simulink model "Assemble_Blocks_May_7_2020"  (R2020a)
settings: Solver=VariableStepAuto  StartTime=0.0  StopTime=100  RelTol=1e-3
libraries: sailbot_library x19
settings Model: Creator=tylerlum  LastModifiedBy=Nicolas
settings SFSimCC: CustomCodeUndefinedFunction=UseInterfaceOnly

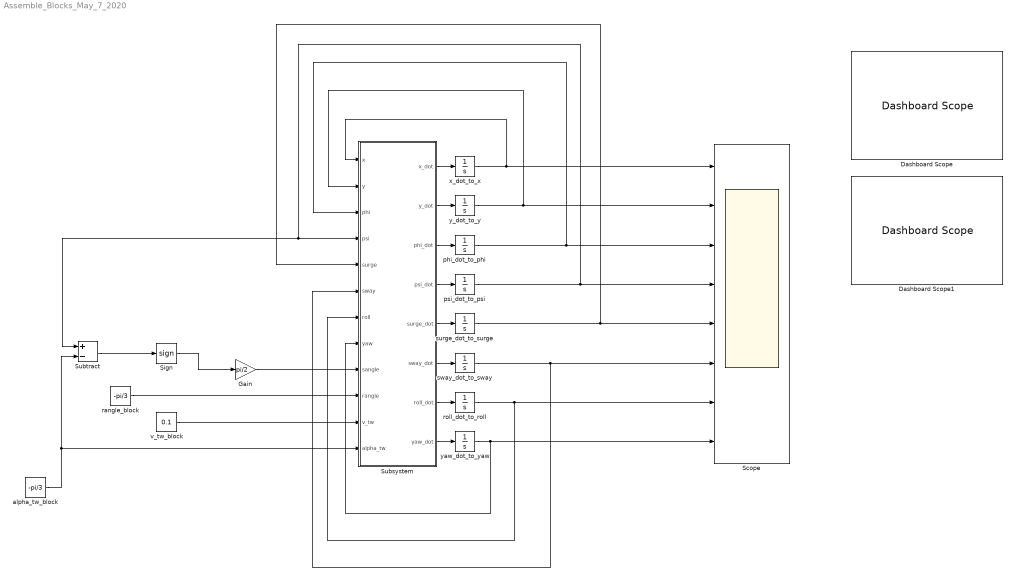
== system Assemble_Blocks_May_7_2020 ==
  Dashboard Scope : DashboardScope
  Dashboard Scope1 : DashboardScope
  Gain : Gain  Gain=pi/2
  Scope : Scope  NumInputPorts=8
  Sign : Signum
  Subsystem : Subsystem
  Subtract : Sum  Inputs=+-
  alpha_tw_block : Constant  Value=-pi/3
  phi_dot_to_phi : Integrator
  psi_dot_to_psi : Integrator  InitialCondition=pi/2
  rangle_block : Constant  Value=-pi/3
  roll_dot_to_roll : Integrator
  surge_dot_to_surge : Integrator
  sway_dot_to_sway : Integrator
  v_tw_block : Constant  Value=0.1
  x_dot_to_x : Integrator
  y_dot_to_y : Integrator
  yaw_dot_to_yaw : Integrator
  wires:
  Subsystem/1(x_dot) -> x_dot_to_x/1
  x_dot_to_x/1 -> Scope/1, Subsystem/1(x)
  Subsystem/2(y_dot) -> y_dot_to_y/1
  Subsystem/3(phi_dot) -> phi_dot_to_phi/1
  Subsystem/4(psi_dot) -> psi_dot_to_psi/1
  Subsystem/5(surge_dot) -> surge_dot_to_surge/1
  Subsystem/6(sway_dot) -> sway_dot_to_sway/1
  Subsystem/7(roll_dot) -> roll_dot_to_roll/1
  Subsystem/8(yaw_dot) -> yaw_dot_to_yaw/1
  y_dot_to_y/1 -> Scope/2, Subsystem/2(y)
  phi_dot_to_phi/1 -> Subsystem/3(phi), Scope/3
  psi_dot_to_psi/1 -> Subsystem/4(psi), Subtract/1, Scope/4
  yaw_dot_to_yaw/1 -> Scope/8, Subsystem/8(yaw)
  roll_dot_to_roll/1 -> Scope/7, Subsystem/7(roll)
  sway_dot_to_sway/1 -> Scope/6, Subsystem/6(sway)
  surge_dot_to_surge/1 -> Subsystem/5(surge), Scope/5
  rangle_block/1 -> Subsystem/10(rangle)
  v_tw_block/1 -> Subsystem/11(v_tw)
  alpha_tw_block/1 -> Subsystem/12(alpha_tw), Subtract/2
  Gain/1 -> Subsystem/9(sangle)
  Subtract/1 -> Sign/1
  Sign/1 -> Gain/1

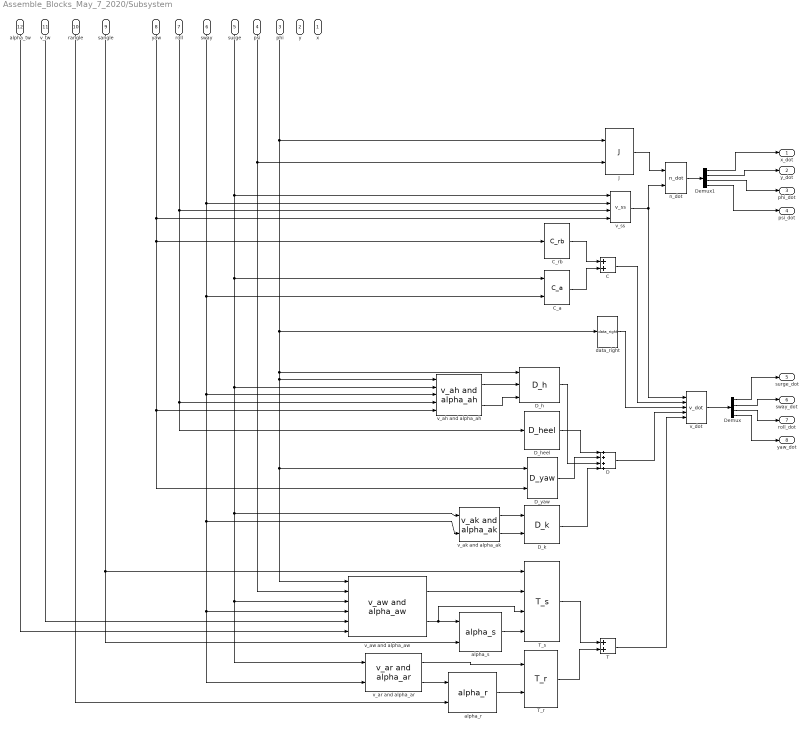
== system Assemble_Blocks_May_7_2020/Subsystem ==
  x : Inport
  y : Inport  Port=2
  phi : Inport  Port=3
  psi : Inport  Port=4
  surge : Inport  Port=5
  sway : Inport  Port=6
  roll : Inport  Port=7
  yaw : Inport  Port=8
  sangle : Inport  Port=9
  rangle : Inport  Port=10
  v_tw : Inport  Port=11
  alpha_tw : Inport  Port=12
  C : Sum
  C_a : sailbot_library/C_a  SystemSampleTime=-1  Latency=0  AutoFrameSizeCalculation=off
  C_rb : sailbot_library/C_rb  SystemSampleTime=-1  Latency=0  AutoFrameSizeCalculation=off
  D : Sum  Inputs=4
  D_h : sailbot_library/D_h  SystemSampleTime=-1  Latency=0  AutoFrameSizeCalculation=off
  "D_heel " : sailbot_library/D_heel   SystemSampleTime=-1  Latency=0  AutoFrameSizeCalculation=off
  D_k : sailbot_library/D_k  SystemSampleTime=-1  Latency=0  AutoFrameSizeCalculation=off
  D_yaw : sailbot_library/D_yaw  SystemSampleTime=-1  Latency=0  AutoFrameSizeCalculation=off
  Demux : Demux
  Demux1 : Demux
  J : sailbot_library/J  SystemSampleTime=-1  Latency=0  AutoFrameSizeCalculation=off
  T : Sum
  T_r : sailbot_library/T_r  SystemSampleTime=-1  Latency=0  AutoFrameSizeCalculation=off
  "T_s " : sailbot_library/T_s   SystemSampleTime=-1  Latency=0  AutoFrameSizeCalculation=off
  alpha_r : sailbot_library/alpha_r  SystemSampleTime=-1  Latency=0  AutoFrameSizeCalculation=off
  alpha_s : sailbot_library/alpha_s  SystemSampleTime=-1  Latency=0  AutoFrameSizeCalculation=off
  data_right : sailbot_library/data_right  SystemSampleTime=-1  Latency=0  AutoFrameSizeCalculation=off
  n_dot : sailbot_library/n_dot  SystemSampleTime=-1  Latency=0  AutoFrameSizeCalculation=off
  v_ah and alpha_ah : sailbot_library/v_ah and alpha_ah  SystemSampleTime=-1  Latency=0  AutoFrameSizeCalculation=off
  v_ak and alpha_ak : sailbot_library/v_ak and alpha_ak  SystemSampleTime=-1  Latency=0  AutoFrameSizeCalculation=off
  v_ar and alpha_ar : sailbot_library/v_ar and alpha_ar  SystemSampleTime=-1  Latency=0  AutoFrameSizeCalculation=off
  v_aw and alpha_aw : sailbot_library/v_aw and alpha_aw  SystemSampleTime=-1  Latency=0  AutoFrameSizeCalculation=off
  v_dot : sailbot_library/v_dot  SystemSampleTime=-1  Latency=0  AutoFrameSizeCalculation=off
  v_ss : sailbot_library/v_ss  SystemSampleTime=-1  Latency=0  AutoFrameSizeCalculation=off
  x_dot : Outport  VectorParamsAs1DForOutWhenUnconnected=off
  y_dot : Outport  Port=2  VectorParamsAs1DForOutWhenUnconnected=off
  phi_dot : Outport  Port=3  VectorParamsAs1DForOutWhenUnconnected=off
  psi_dot : Outport  Port=4  VectorParamsAs1DForOutWhenUnconnected=off
  surge_dot : Outport  Port=5  VectorParamsAs1DForOutWhenUnconnected=off
  sway_dot : Outport  Port=6  VectorParamsAs1DForOutWhenUnconnected=off
  roll_dot : Outport  Port=7  VectorParamsAs1DForOutWhenUnconnected=off
  yaw_dot : Outport  Port=8  VectorParamsAs1DForOutWhenUnconnected=off
  wires:
  alpha_s/1 -> "T_s "/4
  Demux/4 -> yaw_dot/1
  C/1 -> v_dot/2
  v_ah and alpha_ah/1 -> D_h/2
  D/1 -> v_dot/4
  v_aw and alpha_aw/1 -> "T_s "/2
  v_ak and alpha_ak/1 -> D_k/1
  v_ak and alpha_ak/2 -> D_k/2
  Demux/3 -> roll_dot/1
  C_a/1 -> C/2
  J/1 -> n_dot/1
  psi/1 -> v_aw and alpha_aw/2, J/2
  Demux1/4 -> psi_dot/1
  Demux1/2 -> y_dot/1
  T/1 -> v_dot/5
  v_aw and alpha_aw/2 -> "T_s "/3, alpha_s/1
  sway/1 -> v_ss/2, C_a/2, v_ah and alpha_ah/3, v_aw and alpha_aw/4, v_ar and alpha_ar/2, v_ak and alpha_ak/2
  alpha_r/1 -> T_r/2
  data_right/1 -> v_dot/3
  C_rb/1 -> C/1
  v_ah and alpha_ah/2 -> D_h/3
  v_ss/1 -> v_dot/1, n_dot/2
  n_dot/1 -> Demux1/1
  Demux1/3 -> phi_dot/1
  surge/1 -> v_ak and alpha_ak/1, v_aw and alpha_aw/3, v_ar and alpha_ar/1, v_ah and alpha_ah/2, C_a/1, v_ss/1
  Demux1/1 -> x_dot/1
  v_ar and alpha_ar/1 -> T_r/1
  rangle/1 -> alpha_r/2
  yaw/1 -> v_ss/4, D_yaw/2, v_ah and alpha_ah/5, C_rb/1
  phi/1 -> J/1, data_right/1, D_h/1, D_yaw/1, v_aw and alpha_aw/1, v_ah and alpha_ah/1
  Demux/1 -> surge_dot/1
  sangle/1 -> "T_s "/1, alpha_s/2
  v_ar and alpha_ar/2 -> alpha_r/1
  Demux/2 -> sway_dot/1
  roll/1 -> v_ss/3, v_ah and alpha_ah/4, "D_heel "/1
  v_dot/1 -> Demux/1
  "D_heel "/1 -> D/1
  D_yaw/1 -> D/2
  D_h/1 -> D/3
  D_k/1 -> D/4
  T_r/1 -> T/2
  "T_s "/1 -> T/1
  v_tw/1 -> v_aw and alpha_aw/5
  alpha_tw/1 -> v_aw and alpha_aw/6
